simulink model "t3p33"  (R2013b)
settings: Solver=ode45  StartTime=0.0  StopTime=10  RelTol=1e-3
values from neighbouring files (symbols this model uses):
  c = 1e-6    (= 1e-06)    [practica1t.m]    (also in practica2t.m; t3p3.m = 0.04)
  l = 2.5    [t3p3.m]
  r1 = 10    [t3p3.m]
  r2 = 100    [t3p3.m]
  r3 = 20    [t3p3.m]
settings Model: Creator=xmax1946  LastModifiedBy=xmax1946

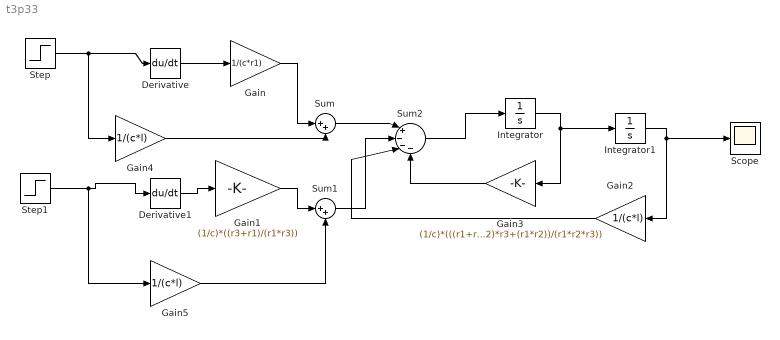
== system t3p33 ==
  Derivative : Derivative
  Derivative1 : Derivative
  Gain : Gain  Gain=1/(c*r1)
  Gain1 : Gain  Gain=(1/c)*((r3+r1)/(r1*r3))
  Gain2 : Gain  Gain=1/(c*l)
  Gain3 : Gain  Gain=(1/c)*(((r1+r2)*r3+(r1*r2))/(r1*r2*r3))
  Gain4 : Gain  Gain=1/(c*l)
  Gain5 : Gain  Gain=1/(c*l)
  Integrator : Integrator
  Integrator1 : Integrator
  Scope : Scope
  Step : Step  SampleTime=0
  Step1 : Step  Time=5  After=.5  SampleTime=0
  Sum : Sum  Inputs=|++
  Sum1 : Sum  Inputs=|++
  Sum2 : Sum  Inputs=|+---
  wires:
  Step/1 -> Gain4/1, Derivative/1
  Derivative/1 -> Gain/1
  Gain/1 -> Sum/1
  Step1/1 -> Gain5/1, Derivative1/1
  Derivative1/1 -> Gain1/1
  Gain1/1 -> Sum1/1
  Sum/1 -> Sum2/1
  Sum1/1 -> Sum2/2
  Sum2/1 -> Integrator/1
  Integrator1/1 -> Scope/1, Gain2/1
  Gain2/1 -> Sum2/3
  Integrator/1 -> Gain3/1, Integrator1/1
  Gain3/1 -> Sum2/4
  Gain4/1 -> Sum/2
  Gain5/1 -> Sum1/2
